simulink model "consigna_5_1"  (R2024b)
settings: Solver=VariableStepAuto  StartTime=0.0  StopTime=1  MaxStep=1e-4  RelTol=1e-3
InitFcn:
  | parametros
undefined symbols (not defined in the file or in its folder): alpha_cu, b_eq, b_l, b_m, C_ts, J_eq, J_l, J_m, k_l, L_d, L_ls, L_q, lambda_m, P_p, r, R_s_40, R_ts_amb, Temp_s_ref
(part 2 of 3)

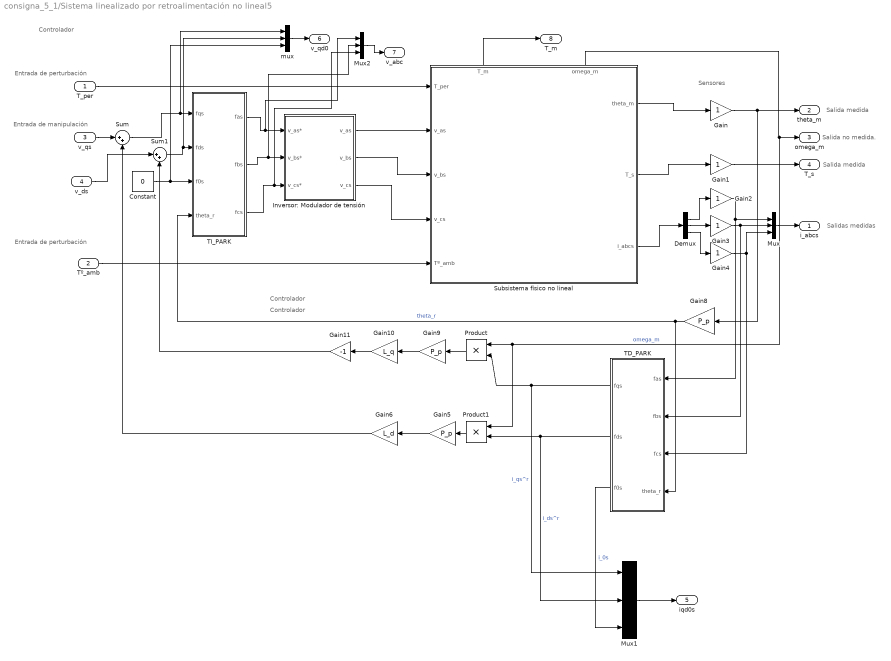
== system consigna_5_1/Sistema linealizado por retroalimentación no lineal5 ==
  note: Entrada de perturbación
  note: Entrada de manipulación
  note: Entrada de perturbación
  note: Controlador
  note: Salida medida
  note: Controlador
  note: Sensores
  note: Salida medida
  note: Salidas medidas
  note: Salida no medida.
  note: Controlador
  T_per : Inport
  Tº_amb : Inport  Port=2
  v_qs : Inport  Port=3
  v_ds : Inport  Port=4
  Constant : Constant  Value=0
  Demux : Demux  Outputs=3
  Gain{,1..4} (5 alike) : Gain
  Gain10 : Gain  Gain=L_q
  Gain11 : Gain  Gain=-1
  Gain5 : Gain  Gain=P_p
  Gain6 : Gain  Gain=L_d
  Gain8 : Gain  Gain=P_p
  Gain9 : Gain  Gain=P_p
  Inversor: Modulador de tensión : Subsystem
  Mux : Mux  Inputs=3
  Mux1 : Mux  Inputs=3
  Mux2 : Mux  Inputs=3
  Product : Product
  Product1 : Product
  Subsistema físico no lineal : Subsystem
      settings: PortSchema="{\"entries\":[{\"content\":{\"sides\":[{\"content\":{\"connectorIds\":[\"In1\",\"In2\",\"In3\",\"In4\",\"In5\"]},\"type\":\"ConnectorPlacement.EquallySpacedRectSide\",\"uuid\":\"67117692-d9ee-40bf-88b2-d8f6a60dc3b5\"},{\"content\":{\"connectorIds\":[\"Out1\",\"Out2\",\"Out3\"],\"side\":\"RIGHT\"},\"type\":\"ConnectorPlacement.EquallySpacedRectSide\",\"uuid\":\"ca2dbe86-e86f-47c7-8eac-1e82e6a5dbc0\"},{\"content\":{\"connectorIds\":[\"Out4\",\"Out5\"],\"side\":\"TOP\"},\"type\":\"ConnectorPlacement.EquallySpacedRectSide\",\"uuid\":\"fbd4a5c3-5162-48dd-8002-932f8e6631f6\"}]},\"type\":\"ConnectorPlacement.EquallySpacedConnector\",\"uuid\":\"e55c07f0-88b9-4508-920f-2bf50421126b\"}],\"packageUris\":[\"http://schema.mathworks.com/mf0/Connector/R2020b\"],\"version\":\"1.0\"}"
  Sum : Sum  Inputs=|++
  Sum1 : Sum  Inputs=|++
  TD_PARK : MATLAB Function  TreatAsAtomicUnit=on
  TI_PARK : MATLAB Function  TreatAsAtomicUnit=on
  mux : Mux  Inputs=3
  i_abcs : Outport
  theta_m : Outport  Port=2
  omega_m : Outport  Port=3
  T_s : Outport  Port=4
  iqd0s : Outport  Port=5
  v_qd0 : Outport  Port=6
  v_abc : Outport  Port=7
  T_m : Outport  Port=8
  wires:
  T_per/1 -> Subsistema físico no lineal/1(T_per)
  Subsistema físico no lineal/2(T_s) -> Gain1/1
  Subsistema físico no lineal/1(theta_m) -> Gain/1
  Tº_amb/1 -> Subsistema físico no lineal/5(Tº_amb)
  Demux/3 -> Gain4/1
  Demux/1 -> Gain2/1
  Gain2/1 -> Mux/1, TD_PARK/1(fas)
  Gain3/1 -> Mux/2, TD_PARK/2(fbs)
  Gain4/1 -> Mux/3, TD_PARK/3(fcs)
  Mux/1 -> i_abcs/1
  Gain/1 -> Gain8/1, theta_m/1
  Subsistema físico no lineal/5(omega_m) -> omega_m/1, Product1/1, Product/1  "omega_m"
  Gain1/1 -> T_s/1
  Gain8/1 -> TI_PARK/4(theta_r), TD_PARK/4(theta_r)  "theta_r"
  TD_PARK/1(fqs) -> Mux1/1, Product/2  "i_qs^r"
  Product/1 -> Gain9/1
  Gain9/1 -> Gain10/1
  Gain10/1 -> Gain11/1
  Constant/1 -> TI_PARK/3(f0s), mux/3
  Inversor: Modulador de tensión/1(v_as) -> Subsistema físico no lineal/2(v_as)
  Inversor: Modulador de tensión/2(v_bs) -> Subsistema físico no lineal/3(v_bs)
  Inversor: Modulador de tensión/3(v_cs) -> Subsistema físico no lineal/4(v_cs)
  TI_PARK/1(fas) -> Mux2/1, Inversor: Modulador de tensión/1(v_as*)
  TI_PARK/2(fbs) -> Mux2/2, Inversor: Modulador de tensión/2(v_bs*)
  TI_PARK/3(fcs) -> Mux2/3, Inversor: Modulador de tensión/3(v_cs*)
  TD_PARK/2(fds) -> Mux1/2, Product1/2  "i_ds^r"
  TD_PARK/3(f0s) -> Mux1/3  "i_0s"
  v_qs/1 -> Sum/1
  Sum/1 -> mux/1, TI_PARK/1(fqs)
  Product1/1 -> Gain5/1
  Gain5/1 -> Gain6/1
  Gain6/1 -> Sum/2
  Mux1/1 -> iqd0s/1
  mux/1 -> v_qd0/1
  Mux2/1 -> v_abc/1
  Subsistema físico no lineal/4(T_m) -> T_m/1
  Subsistema físico no lineal/3(i_abcs) -> Demux/1
  Demux/2 -> Gain3/1
  Gain11/1 -> Sum1/2
  v_ds/1 -> Sum1/1
  Sum1/1 -> mux/2, TI_PARK/2(fds)

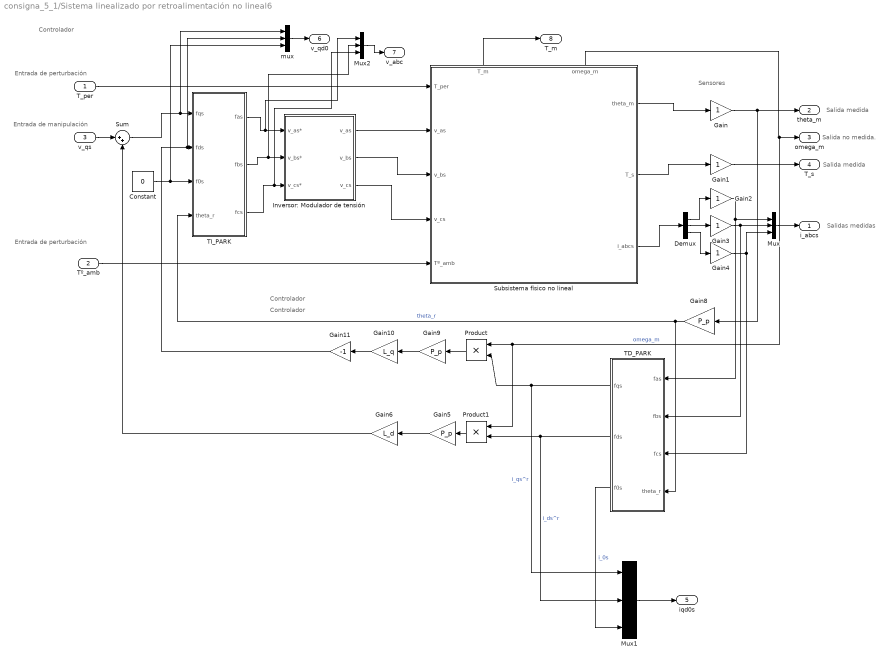
== system consigna_5_1/Sistema linealizado por retroalimentación no lineal6 ==
  note: Entrada de perturbación
  note: Entrada de manipulación
  note: Entrada de perturbación
  note: Controlador
  note: Salida medida
  note: Controlador
  note: Sensores
  note: Salida medida
  note: Salidas medidas
  note: Salida no medida.
  note: Controlador
  T_per : Inport
  Tº_amb : Inport  Port=2
  v_qs : Inport  Port=3
  Constant : Constant  Value=0
  Demux : Demux  Outputs=3
  Gain{,1..4} (5 alike) : Gain
  Gain10 : Gain  Gain=L_q
  Gain11 : Gain  Gain=-1
  Gain5 : Gain  Gain=P_p
  Gain6 : Gain  Gain=L_d
  Gain8 : Gain  Gain=P_p
  Gain9 : Gain  Gain=P_p
  Inversor: Modulador de tensión : Subsystem
  Mux : Mux  Inputs=3
  Mux1 : Mux  Inputs=3
  Mux2 : Mux  Inputs=3
  Product : Product
  Product1 : Product
  Subsistema físico no lineal : Subsystem
      settings: PortSchema="{\"entries\":[{\"content\":{\"sides\":[{\"content\":{\"connectorIds\":[\"In1\",\"In2\",\"In3\",\"In4\",\"In5\"]},\"type\":\"ConnectorPlacement.EquallySpacedRectSide\",\"uuid\":\"67117692-d9ee-40bf-88b2-d8f6a60dc3b5\"},{\"content\":{\"connectorIds\":[\"Out1\",\"Out2\",\"Out3\"],\"side\":\"RIGHT\"},\"type\":\"ConnectorPlacement.EquallySpacedRectSide\",\"uuid\":\"ca2dbe86-e86f-47c7-8eac-1e82e6a5dbc0\"},{\"content\":{\"connectorIds\":[\"Out4\",\"Out5\"],\"side\":\"TOP\"},\"type\":\"ConnectorPlacement.EquallySpacedRectSide\",\"uuid\":\"fbd4a5c3-5162-48dd-8002-932f8e6631f6\"}]},\"type\":\"ConnectorPlacement.EquallySpacedConnector\",\"uuid\":\"e55c07f0-88b9-4508-920f-2bf50421126b\"}],\"packageUris\":[\"http://schema.mathworks.com/mf0/Connector/R2020b\"],\"version\":\"1.0\"}"
  Sum : Sum  Inputs=|++
  TD_PARK : MATLAB Function  TreatAsAtomicUnit=on
  TI_PARK : MATLAB Function  TreatAsAtomicUnit=on
  mux : Mux  Inputs=3
  i_abcs : Outport
  theta_m : Outport  Port=2
  omega_m : Outport  Port=3
  T_s : Outport  Port=4
  iqd0s : Outport  Port=5
  v_qd0 : Outport  Port=6
  v_abc : Outport  Port=7
  T_m : Outport  Port=8
  wires:
  T_per/1 -> Subsistema físico no lineal/1(T_per)
  Subsistema físico no lineal/2(T_s) -> Gain1/1
  Subsistema físico no lineal/1(theta_m) -> Gain/1
  Tº_amb/1 -> Subsistema físico no lineal/5(Tº_amb)
  Demux/3 -> Gain4/1
  Demux/1 -> Gain2/1
  Gain2/1 -> Mux/1, TD_PARK/1(fas)
  Gain3/1 -> Mux/2, TD_PARK/2(fbs)
  Gain4/1 -> Mux/3, TD_PARK/3(fcs)
  Mux/1 -> i_abcs/1
  Gain/1 -> Gain8/1, theta_m/1
  Subsistema físico no lineal/5(omega_m) -> omega_m/1, Product1/1, Product/1  "omega_m"
  Gain1/1 -> T_s/1
  Gain8/1 -> TI_PARK/4(theta_r), TD_PARK/4(theta_r)  "theta_r"
  TD_PARK/1(fqs) -> Mux1/1, Product/2  "i_qs^r"
  Product/1 -> Gain9/1
  Gain9/1 -> Gain10/1
  Gain11/1 -> mux/2, TI_PARK/2(fds)
  Gain10/1 -> Gain11/1
  Constant/1 -> TI_PARK/3(f0s), mux/3
  Inversor: Modulador de tensión/1(v_as) -> Subsistema físico no lineal/2(v_as)
  Inversor: Modulador de tensión/2(v_bs) -> Subsistema físico no lineal/3(v_bs)
  Inversor: Modulador de tensión/3(v_cs) -> Subsistema físico no lineal/4(v_cs)
  TI_PARK/1(fas) -> Mux2/1, Inversor: Modulador de tensión/1(v_as*)
  TI_PARK/2(fbs) -> Mux2/2, Inversor: Modulador de tensión/2(v_bs*)
  TI_PARK/3(fcs) -> Mux2/3, Inversor: Modulador de tensión/3(v_cs*)
  TD_PARK/2(fds) -> Mux1/2, Product1/2  "i_ds^r"
  TD_PARK/3(f0s) -> Mux1/3  "i_0s"
  v_qs/1 -> Sum/1
  Sum/1 -> mux/1, TI_PARK/1(fqs)
  Product1/1 -> Gain5/1
  Gain5/1 -> Gain6/1
  Gain6/1 -> Sum/2
  Mux1/1 -> iqd0s/1
  mux/1 -> v_qd0/1
  Mux2/1 -> v_abc/1
  Subsistema físico no lineal/4(T_m) -> T_m/1
  Subsistema físico no lineal/3(i_abcs) -> Demux/1
  Demux/2 -> Gain3/1

== system consigna_5_1/Sistema completo/Subsistema físico no lineal ==
  note: Retroalimentación natural del torque gravitacional
  Tº_amb : Inport
  v_as : Inport  Port=2
  v_bs : Inport  Port=3
  v_cs : Inport  Port=4
  T_per : Inport  Port=5
  Gain : Gain  Gain=P_p
  Gain1 : Gain  Gain=1/r
  Gain2 : Gain  Gain=k_l
  Mux : Mux  Inputs=3
  Sin : Trigonometry
  Subsistema electromagnético : Subsystem
      settings: PortSchema="{\"entries\":[{\"content\":{\"sides\":[{\"content\":{\"connectorIds\":[\"In1\",\"In2\",\"In3\",\"In4\"]},\"type\":\"ConnectorPlacement.EquallySpacedRectSide\",\"uuid\":\"c9fae60f-a644-4c7d-9a50-e330e891aba8\"},{\"content\":{\"connectorIds\":[\"Out1\",\"Out2\",\"Out3\",\"Out4\"],\"side\":\"RIGHT\"},\"type\":\"ConnectorPlacement.EquallySpacedRectSide\",\"uuid\":\"1bd25713-f5e9-4106-83eb-fb9f8a30d88e\"},{\"content\":{\"connectorIds\":[\"In5\"],\"side\":\"TOP\"},\"type\":\"ConnectorPlacement.EquallySpacedRectSide\",\"uuid\":\"c2f005dd-e04f-426d-b804-ce475aa5422d\"}]},\"type\":\"ConnectorPlacement.EquallySpacedConnector\",\"uuid\":\"9bdc4406-fcef-47cb-a5c0-d4f33f547a91\"}],\"packageUris\":[\"http://schema.mathworks.com/mf0/Connector/R2020b\"],\"version\":\"1.0\"}"
  Subsistema mecánico completo : Subsystem
  Subsistema térmico : Subsystem
  Sum : Sum  Inputs=++|
  TD_PARK : MATLAB Function  TreatAsAtomicUnit=on
  TI_PARK : MATLAB Function  TreatAsAtomicUnit=on
  theta_m : Outport
  omega_m : Outport  Port=2
  T_s : Outport  Port=3
  i_abcs : Outport  Port=4
  wires:
  Subsistema electromagnético/4(T_m) -> Subsistema mecánico completo/1(T_m)
  Subsistema electromagnético/3(i_0s) -> Subsistema térmico/3(i_0s^r), TI_PARK/3(f0s)
  Subsistema mecánico completo/2(omega_m(t)) -> Subsistema electromagnético/5(omega_m), omega_m/1
  Subsistema electromagnético/1(i_qs^r) -> Subsistema térmico/1(i_qs^r), TI_PARK/1(fqs)
  Subsistema electromagnético/2(i_ds^r) -> Subsistema térmico/2(i_ds^r), TI_PARK/2(fds)
  Sum/1 -> Subsistema mecánico completo/2(T_l)  "T_l"
  TD_PARK/1(fqs) -> Subsistema electromagnético/1(v_qs^r)
  Subsistema mecánico completo/1(theta_m(t)) -> theta_m/1, Gain1/1, Gain/1
  Tº_amb/1 -> Subsistema térmico/4(Tº_amb)
  Mux/1 -> i_abcs/1
  TI_PARK/1(fas) -> Mux/1
  TI_PARK/2(fbs) -> Mux/2
  TI_PARK/3(fcs) -> Mux/3
  v_as/1 -> TD_PARK/1(fas)
  v_cs/1 -> TD_PARK/3(fcs)
  Gain/1 -> TI_PARK/4(theta_r), TD_PARK/4(theta_r)
  v_bs/1 -> TD_PARK/2(fbs)
  Gain1/1 -> Sin/1
  Sin/1 -> Gain2/1
  Gain2/1 -> Sum/1
  T_per/1 -> Sum/2
  TD_PARK/2(fds) -> Subsistema electromagnético/2(v_ds^r)
  TD_PARK/3(f0s) -> Subsistema electromagnético/3(v_0s)
  Subsistema térmico/1(r_s) -> Subsistema electromagnético/4(r_s)
  Subsistema térmico/2(T_s) -> T_s/1

== system consigna_5_1/Sistema linealizado por retroalimentación no lineal1/Inversor: Modulador de tensión ==
  v_as* : Inport
  v_bs* : Inport  Port=2
  v_cs* : Inport  Port=3
  Gain5 : Gain
  Gain6 : Gain
  Gain7 : Gain
  v_as : Outport
  v_bs : Outport  Port=2
  v_cs : Outport  Port=3
  wires:
  v_as*/1 -> Gain5/1
  Gain5/1 -> v_as/1
  v_cs*/1 -> Gain7/1
  v_bs*/1 -> Gain6/1
  Gain7/1 -> v_cs/1
  Gain6/1 -> v_bs/1

== system consigna_5_1/Sistema linealizado por retroalimentación no lineal1/Subsistema físico no lineal ==
  note: Retroalimentación natural del torque gravitacional
  T_per : Inport
  v_as : Inport  Port=2
  v_bs : Inport  Port=3
  v_cs : Inport  Port=4
  Tº_amb : Inport  Port=5
  Gain : Gain  Gain=P_p
  Gain1 : Gain  Gain=1/r
  Gain2 : Gain  Gain=k_l
  Mux : Mux  Inputs=3
  Scope : Scope
  Sin : Trigonometry
  Subsistema electromagnético : Subsystem
      settings: PortSchema="{\"entries\":[{\"content\":{\"sides\":[{\"content\":{\"connectorIds\":[\"In1\",\"In2\",\"In3\",\"In4\"]},\"type\":\"ConnectorPlacement.EquallySpacedRectSide\",\"uuid\":\"c9fae60f-a644-4c7d-9a50-e330e891aba8\"},{\"content\":{\"connectorIds\":[\"Out1\",\"Out2\",\"Out3\",\"Out4\"],\"side\":\"RIGHT\"},\"type\":\"ConnectorPlacement.EquallySpacedRectSide\",\"uuid\":\"1bd25713-f5e9-4106-83eb-fb9f8a30d88e\"},{\"content\":{\"connectorIds\":[\"In5\"],\"side\":\"TOP\"},\"type\":\"ConnectorPlacement.EquallySpacedRectSide\",\"uuid\":\"c2f005dd-e04f-426d-b804-ce475aa5422d\"}]},\"type\":\"ConnectorPlacement.EquallySpacedConnector\",\"uuid\":\"9bdc4406-fcef-47cb-a5c0-d4f33f547a91\"}],\"packageUris\":[\"http://schema.mathworks.com/mf0/Connector/R2020b\"],\"version\":\"1.0\"}"
  Subsistema mecánico completo : Subsystem
  Subsistema térmico : Subsystem
  Sum : Sum  Inputs=++|
  TD_PARK : MATLAB Function  TreatAsAtomicUnit=on
  TI_PARK : MATLAB Function  TreatAsAtomicUnit=on
  theta_m : Outport
  T_s : Outport  Port=2
  i_abcs : Outport  Port=3
  T_m : Outport  Port=4
  omega_m : Outport  Port=5
  wires:
  Subsistema electromagnético/4(T_m) -> T_m/1, Subsistema mecánico completo/1(T_m)
  Subsistema electromagnético/3(i_0s) -> Subsistema térmico/3(i_0s^r), TI_PARK/3(f0s)
  Subsistema mecánico completo/2(omega_m(t)) -> Subsistema electromagnético/5(omega_m), Scope/1, omega_m/1
  Subsistema electromagnético/1(i_qs^r) -> Subsistema térmico/1(i_qs^r), TI_PARK/1(fqs)
  Subsistema electromagnético/2(i_ds^r) -> Subsistema térmico/2(i_ds^r), TI_PARK/2(fds)
  Sum/1 -> Subsistema mecánico completo/2(T_l)  "T_l"
  TD_PARK/1(fqs) -> Subsistema electromagnético/1(v_qs^r)
  Tº_amb/1 -> Subsistema térmico/4(Tº_amb)
  Mux/1 -> i_abcs/1
  TI_PARK/1(fas) -> Mux/1
  TI_PARK/2(fbs) -> Mux/2
  TI_PARK/3(fcs) -> Mux/3
  v_as/1 -> TD_PARK/1(fas)
  v_cs/1 -> TD_PARK/3(fcs)
  Gain/1 -> TI_PARK/4(theta_r), TD_PARK/4(theta_r)
  v_bs/1 -> TD_PARK/2(fbs)
  Gain1/1 -> Sin/1
  Sin/1 -> Gain2/1
  Gain2/1 -> Sum/1
  T_per/1 -> Sum/2
  TD_PARK/2(fds) -> Subsistema electromagnético/2(v_ds^r)
  TD_PARK/3(f0s) -> Subsistema electromagnético/3(v_0s)
  Subsistema térmico/1(r_s) -> Subsistema electromagnético/4(r_s)
  Subsistema térmico/2(T_s) -> T_s/1
  Subsistema mecánico completo/1(theta_m(t)) -> theta_m/1, Gain1/1, Gain/1

== system consigna_5_1/Sistema linealizado por retroalimentación no lineal2/Inversor: Modulador de tensión ==
  v_as* : Inport
  v_bs* : Inport  Port=2
  v_cs* : Inport  Port=3
  Gain5 : Gain
  Gain6 : Gain
  Gain7 : Gain
  v_as : Outport
  v_bs : Outport  Port=2
  v_cs : Outport  Port=3
  wires:
  v_as*/1 -> Gain5/1
  Gain5/1 -> v_as/1
  v_cs*/1 -> Gain7/1
  v_bs*/1 -> Gain6/1
  Gain7/1 -> v_cs/1
  Gain6/1 -> v_bs/1

== system consigna_5_1/Sistema linealizado por retroalimentación no lineal2/Subsistema físico no lineal ==
  note: Retroalimentación natural del torque gravitacional
  T_per : Inport
  v_as : Inport  Port=2
  v_bs : Inport  Port=3
  v_cs : Inport  Port=4
  Tº_amb : Inport  Port=5
  Gain : Gain  Gain=P_p
  Gain1 : Gain  Gain=1/r
  Gain2 : Gain  Gain=k_l
  Mux : Mux  Inputs=3
  Scope : Scope
  Sin : Trigonometry
  Subsistema electromagnético : Subsystem
      settings: PortSchema="{\"entries\":[{\"content\":{\"sides\":[{\"content\":{\"connectorIds\":[\"In1\",\"In2\",\"In3\",\"In4\"]},\"type\":\"ConnectorPlacement.EquallySpacedRectSide\",\"uuid\":\"c9fae60f-a644-4c7d-9a50-e330e891aba8\"},{\"content\":{\"connectorIds\":[\"Out1\",\"Out2\",\"Out3\",\"Out4\"],\"side\":\"RIGHT\"},\"type\":\"ConnectorPlacement.EquallySpacedRectSide\",\"uuid\":\"1bd25713-f5e9-4106-83eb-fb9f8a30d88e\"},{\"content\":{\"connectorIds\":[\"In5\"],\"side\":\"TOP\"},\"type\":\"ConnectorPlacement.EquallySpacedRectSide\",\"uuid\":\"c2f005dd-e04f-426d-b804-ce475aa5422d\"}]},\"type\":\"ConnectorPlacement.EquallySpacedConnector\",\"uuid\":\"9bdc4406-fcef-47cb-a5c0-d4f33f547a91\"}],\"packageUris\":[\"http://schema.mathworks.com/mf0/Connector/R2020b\"],\"version\":\"1.0\"}"
  Subsistema mecánico completo : Subsystem
  Subsistema térmico : Subsystem
  Sum : Sum  Inputs=++|
  TD_PARK : MATLAB Function  TreatAsAtomicUnit=on
  TI_PARK : MATLAB Function  TreatAsAtomicUnit=on
  theta_m : Outport
  T_s : Outport  Port=2
  i_abcs : Outport  Port=3
  T_m : Outport  Port=4
  omega_m : Outport  Port=5
  wires:
  Subsistema electromagnético/4(T_m) -> T_m/1, Subsistema mecánico completo/1(T_m)
  Subsistema electromagnético/3(i_0s) -> Subsistema térmico/3(i_0s^r), TI_PARK/3(f0s)
  Subsistema mecánico completo/2(omega_m(t)) -> Subsistema electromagnético/5(omega_m), Scope/1, omega_m/1
  Subsistema electromagnético/1(i_qs^r) -> Subsistema térmico/1(i_qs^r), TI_PARK/1(fqs)
  Subsistema electromagnético/2(i_ds^r) -> Subsistema térmico/2(i_ds^r), TI_PARK/2(fds)
  Sum/1 -> Subsistema mecánico completo/2(T_l)  "T_l"
  TD_PARK/1(fqs) -> Subsistema electromagnético/1(v_qs^r)
  Tº_amb/1 -> Subsistema térmico/4(Tº_amb)
  Mux/1 -> i_abcs/1
  TI_PARK/1(fas) -> Mux/1
  TI_PARK/2(fbs) -> Mux/2
  TI_PARK/3(fcs) -> Mux/3
  v_as/1 -> TD_PARK/1(fas)
  v_cs/1 -> TD_PARK/3(fcs)
  Gain/1 -> TI_PARK/4(theta_r), TD_PARK/4(theta_r)
  v_bs/1 -> TD_PARK/2(fbs)
  Gain1/1 -> Sin/1
  Sin/1 -> Gain2/1
  Gain2/1 -> Sum/1
  T_per/1 -> Sum/2
  TD_PARK/2(fds) -> Subsistema electromagnético/2(v_ds^r)
  TD_PARK/3(f0s) -> Subsistema electromagnético/3(v_0s)
  Subsistema térmico/1(r_s) -> Subsistema electromagnético/4(r_s)
  Subsistema térmico/2(T_s) -> T_s/1
  Subsistema mecánico completo/1(theta_m(t)) -> theta_m/1, Gain1/1, Gain/1

== system consigna_5_1/Sistema linealizado por retroalimentación no lineal3/Inversor: Modulador de tensión ==
  v_as* : Inport
  v_bs* : Inport  Port=2
  v_cs* : Inport  Port=3
  Gain5 : Gain
  Gain6 : Gain
  Gain7 : Gain
  v_as : Outport
  v_bs : Outport  Port=2
  v_cs : Outport  Port=3
  wires:
  v_as*/1 -> Gain5/1
  Gain5/1 -> v_as/1
  v_cs*/1 -> Gain7/1
  v_bs*/1 -> Gain6/1
  Gain7/1 -> v_cs/1
  Gain6/1 -> v_bs/1

== system consigna_5_1/Sistema linealizado por retroalimentación no lineal3/Subsistema físico no lineal ==
  note: Retroalimentación natural del torque gravitacional
  T_per : Inport
  v_as : Inport  Port=2
  v_bs : Inport  Port=3
  v_cs : Inport  Port=4
  Tº_amb : Inport  Port=5
  Gain : Gain  Gain=P_p
  Gain1 : Gain  Gain=1/r
  Gain2 : Gain  Gain=k_l
  Mux : Mux  Inputs=3
  Scope : Scope
  Sin : Trigonometry
  Subsistema electromagnético : Subsystem
      settings: PortSchema="{\"entries\":[{\"content\":{\"sides\":[{\"content\":{\"connectorIds\":[\"In1\",\"In2\",\"In3\",\"In4\"]},\"type\":\"ConnectorPlacement.EquallySpacedRectSide\",\"uuid\":\"c9fae60f-a644-4c7d-9a50-e330e891aba8\"},{\"content\":{\"connectorIds\":[\"Out1\",\"Out2\",\"Out3\",\"Out4\"],\"side\":\"RIGHT\"},\"type\":\"ConnectorPlacement.EquallySpacedRectSide\",\"uuid\":\"1bd25713-f5e9-4106-83eb-fb9f8a30d88e\"},{\"content\":{\"connectorIds\":[\"In5\"],\"side\":\"TOP\"},\"type\":\"ConnectorPlacement.EquallySpacedRectSide\",\"uuid\":\"c2f005dd-e04f-426d-b804-ce475aa5422d\"}]},\"type\":\"ConnectorPlacement.EquallySpacedConnector\",\"uuid\":\"9bdc4406-fcef-47cb-a5c0-d4f33f547a91\"}],\"packageUris\":[\"http://schema.mathworks.com/mf0/Connector/R2020b\"],\"version\":\"1.0\"}"
  Subsistema mecánico completo : Subsystem
  Subsistema térmico : Subsystem
  Sum : Sum  Inputs=++|
  TD_PARK : MATLAB Function  TreatAsAtomicUnit=on
  TI_PARK : MATLAB Function  TreatAsAtomicUnit=on
  theta_m : Outport
  T_s : Outport  Port=2
  i_abcs : Outport  Port=3
  T_m : Outport  Port=4
  omega_m : Outport  Port=5
  wires:
  Subsistema electromagnético/4(T_m) -> T_m/1, Subsistema mecánico completo/1(T_m)
  Subsistema electromagnético/3(i_0s) -> Subsistema térmico/3(i_0s^r), TI_PARK/3(f0s)
  Subsistema mecánico completo/2(omega_m(t)) -> Subsistema electromagnético/5(omega_m), Scope/1, omega_m/1
  Subsistema electromagnético/1(i_qs^r) -> Subsistema térmico/1(i_qs^r), TI_PARK/1(fqs)
  Subsistema electromagnético/2(i_ds^r) -> Subsistema térmico/2(i_ds^r), TI_PARK/2(fds)
  Sum/1 -> Subsistema mecánico completo/2(T_l)  "T_l"
  TD_PARK/1(fqs) -> Subsistema electromagnético/1(v_qs^r)
  Tº_amb/1 -> Subsistema térmico/4(Tº_amb)
  Mux/1 -> i_abcs/1
  TI_PARK/1(fas) -> Mux/1
  TI_PARK/2(fbs) -> Mux/2
  TI_PARK/3(fcs) -> Mux/3
  v_as/1 -> TD_PARK/1(fas)
  v_cs/1 -> TD_PARK/3(fcs)
  Gain/1 -> TI_PARK/4(theta_r), TD_PARK/4(theta_r)
  v_bs/1 -> TD_PARK/2(fbs)
  Gain1/1 -> Sin/1
  Sin/1 -> Gain2/1
  Gain2/1 -> Sum/1
  T_per/1 -> Sum/2
  TD_PARK/2(fds) -> Subsistema electromagnético/2(v_ds^r)
  TD_PARK/3(f0s) -> Subsistema electromagnético/3(v_0s)
  Subsistema térmico/1(r_s) -> Subsistema electromagnético/4(r_s)
  Subsistema térmico/2(T_s) -> T_s/1
  Subsistema mecánico completo/1(theta_m(t)) -> theta_m/1, Gain1/1, Gain/1

== system consigna_5_1/Sistema linealizado por retroalimentación no lineal4/Inversor: Modulador de tensión ==
  v_as* : Inport
  v_bs* : Inport  Port=2
  v_cs* : Inport  Port=3
  Gain5 : Gain
  Gain6 : Gain
  Gain7 : Gain
  v_as : Outport
  v_bs : Outport  Port=2
  v_cs : Outport  Port=3
  wires:
  v_as*/1 -> Gain5/1
  Gain5/1 -> v_as/1
  v_cs*/1 -> Gain7/1
  v_bs*/1 -> Gain6/1
  Gain7/1 -> v_cs/1
  Gain6/1 -> v_bs/1

== system consigna_5_1/Sistema linealizado por retroalimentación no lineal4/Subsistema físico no lineal ==
  note: Retroalimentación natural del torque gravitacional
  T_per : Inport
  v_as : Inport  Port=2
  v_bs : Inport  Port=3
  v_cs : Inport  Port=4
  Tº_amb : Inport  Port=5
  Gain : Gain  Gain=P_p
  Gain1 : Gain  Gain=1/r
  Gain2 : Gain  Gain=k_l
  Mux : Mux  Inputs=3
  Scope : Scope
  Sin : Trigonometry
  Subsistema electromagnético : Subsystem
      settings: PortSchema="{\"entries\":[{\"content\":{\"sides\":[{\"content\":{\"connectorIds\":[\"In1\",\"In2\",\"In3\",\"In4\"]},\"type\":\"ConnectorPlacement.EquallySpacedRectSide\",\"uuid\":\"c9fae60f-a644-4c7d-9a50-e330e891aba8\"},{\"content\":{\"connectorIds\":[\"Out1\",\"Out2\",\"Out3\",\"Out4\"],\"side\":\"RIGHT\"},\"type\":\"ConnectorPlacement.EquallySpacedRectSide\",\"uuid\":\"1bd25713-f5e9-4106-83eb-fb9f8a30d88e\"},{\"content\":{\"connectorIds\":[\"In5\"],\"side\":\"TOP\"},\"type\":\"ConnectorPlacement.EquallySpacedRectSide\",\"uuid\":\"c2f005dd-e04f-426d-b804-ce475aa5422d\"}]},\"type\":\"ConnectorPlacement.EquallySpacedConnector\",\"uuid\":\"9bdc4406-fcef-47cb-a5c0-d4f33f547a91\"}],\"packageUris\":[\"http://schema.mathworks.com/mf0/Connector/R2020b\"],\"version\":\"1.0\"}"
  Subsistema mecánico completo : Subsystem
  Subsistema térmico : Subsystem
  Sum : Sum  Inputs=++|
  TD_PARK : MATLAB Function  TreatAsAtomicUnit=on
  TI_PARK : MATLAB Function  TreatAsAtomicUnit=on
  theta_m : Outport
  T_s : Outport  Port=2
  i_abcs : Outport  Port=3
  T_m : Outport  Port=4
  omega_m : Outport  Port=5
  wires:
  Subsistema electromagnético/4(T_m) -> T_m/1, Subsistema mecánico completo/1(T_m)
  Subsistema electromagnético/3(i_0s) -> Subsistema térmico/3(i_0s^r), TI_PARK/3(f0s)
  Subsistema mecánico completo/2(omega_m(t)) -> Subsistema electromagnético/5(omega_m), Scope/1, omega_m/1
  Subsistema electromagnético/1(i_qs^r) -> Subsistema térmico/1(i_qs^r), TI_PARK/1(fqs)
  Subsistema electromagnético/2(i_ds^r) -> Subsistema térmico/2(i_ds^r), TI_PARK/2(fds)
  Sum/1 -> Subsistema mecánico completo/2(T_l)  "T_l"
  TD_PARK/1(fqs) -> Subsistema electromagnético/1(v_qs^r)
  Tº_amb/1 -> Subsistema térmico/4(Tº_amb)
  Mux/1 -> i_abcs/1
  TI_PARK/1(fas) -> Mux/1
  TI_PARK/2(fbs) -> Mux/2
  TI_PARK/3(fcs) -> Mux/3
  v_as/1 -> TD_PARK/1(fas)
  v_cs/1 -> TD_PARK/3(fcs)
  Gain/1 -> TI_PARK/4(theta_r), TD_PARK/4(theta_r)
  v_bs/1 -> TD_PARK/2(fbs)
  Gain1/1 -> Sin/1
  Sin/1 -> Gain2/1
  Gain2/1 -> Sum/1
  T_per/1 -> Sum/2
  TD_PARK/2(fds) -> Subsistema electromagnético/2(v_ds^r)
  TD_PARK/3(f0s) -> Subsistema electromagnético/3(v_0s)
  Subsistema térmico/1(r_s) -> Subsistema electromagnético/4(r_s)
  Subsistema térmico/2(T_s) -> T_s/1
  Subsistema mecánico completo/1(theta_m(t)) -> theta_m/1, Gain1/1, Gain/1

== system consigna_5_1/Sistema linealizado por retroalimentación no lineal5/Inversor: Modulador de tensión ==
  v_as* : Inport
  v_bs* : Inport  Port=2
  v_cs* : Inport  Port=3
  Gain5 : Gain
  Gain6 : Gain
  Gain7 : Gain
  v_as : Outport
  v_bs : Outport  Port=2
  v_cs : Outport  Port=3
  wires:
  v_as*/1 -> Gain5/1
  Gain5/1 -> v_as/1
  v_cs*/1 -> Gain7/1
  v_bs*/1 -> Gain6/1
  Gain7/1 -> v_cs/1
  Gain6/1 -> v_bs/1

== system consigna_5_1/Sistema linealizado por retroalimentación no lineal5/Subsistema físico no lineal ==
  note: Retroalimentación natural del torque gravitacional
  T_per : Inport
  v_as : Inport  Port=2
  v_bs : Inport  Port=3
  v_cs : Inport  Port=4
  Tº_amb : Inport  Port=5
  Gain : Gain  Gain=P_p
  Gain1 : Gain  Gain=1/r
  Gain2 : Gain  Gain=k_l
  Mux : Mux  Inputs=3
  Scope : Scope
  Sin : Trigonometry
  Subsistema electromagnético : Subsystem
      settings: PortSchema="{\"entries\":[{\"content\":{\"sides\":[{\"content\":{\"connectorIds\":[\"In1\",\"In2\",\"In3\",\"In4\"]},\"type\":\"ConnectorPlacement.EquallySpacedRectSide\",\"uuid\":\"c9fae60f-a644-4c7d-9a50-e330e891aba8\"},{\"content\":{\"connectorIds\":[\"Out1\",\"Out2\",\"Out3\",\"Out4\"],\"side\":\"RIGHT\"},\"type\":\"ConnectorPlacement.EquallySpacedRectSide\",\"uuid\":\"1bd25713-f5e9-4106-83eb-fb9f8a30d88e\"},{\"content\":{\"connectorIds\":[\"In5\"],\"side\":\"TOP\"},\"type\":\"ConnectorPlacement.EquallySpacedRectSide\",\"uuid\":\"c2f005dd-e04f-426d-b804-ce475aa5422d\"}]},\"type\":\"ConnectorPlacement.EquallySpacedConnector\",\"uuid\":\"9bdc4406-fcef-47cb-a5c0-d4f33f547a91\"}],\"packageUris\":[\"http://schema.mathworks.com/mf0/Connector/R2020b\"],\"version\":\"1.0\"}"
  Subsistema mecánico completo : Subsystem
  Subsistema térmico : Subsystem
  Sum : Sum  Inputs=++|
  TD_PARK : MATLAB Function  TreatAsAtomicUnit=on
  TI_PARK : MATLAB Function  TreatAsAtomicUnit=on
  theta_m : Outport
  T_s : Outport  Port=2
  i_abcs : Outport  Port=3
  T_m : Outport  Port=4
  omega_m : Outport  Port=5
  wires:
  Subsistema electromagnético/4(T_m) -> T_m/1, Subsistema mecánico completo/1(T_m)
  Subsistema electromagnético/3(i_0s) -> Subsistema térmico/3(i_0s^r), TI_PARK/3(f0s)
  Subsistema mecánico completo/2(omega_m(t)) -> Subsistema electromagnético/5(omega_m), Scope/1, omega_m/1
  Subsistema electromagnético/1(i_qs^r) -> Subsistema térmico/1(i_qs^r), TI_PARK/1(fqs)
  Subsistema electromagnético/2(i_ds^r) -> Subsistema térmico/2(i_ds^r), TI_PARK/2(fds)
  Sum/1 -> Subsistema mecánico completo/2(T_l)  "T_l"
  TD_PARK/1(fqs) -> Subsistema electromagnético/1(v_qs^r)
  Tº_amb/1 -> Subsistema térmico/4(Tº_amb)
  Mux/1 -> i_abcs/1
  TI_PARK/1(fas) -> Mux/1
  TI_PARK/2(fbs) -> Mux/2
  TI_PARK/3(fcs) -> Mux/3
  v_as/1 -> TD_PARK/1(fas)
  v_cs/1 -> TD_PARK/3(fcs)
  Gain/1 -> TI_PARK/4(theta_r), TD_PARK/4(theta_r)
  v_bs/1 -> TD_PARK/2(fbs)
  Gain1/1 -> Sin/1
  Sin/1 -> Gain2/1
  Gain2/1 -> Sum/1
  T_per/1 -> Sum/2
  TD_PARK/2(fds) -> Subsistema electromagnético/2(v_ds^r)
  TD_PARK/3(f0s) -> Subsistema electromagnético/3(v_0s)
  Subsistema térmico/1(r_s) -> Subsistema electromagnético/4(r_s)
  Subsistema térmico/2(T_s) -> T_s/1
  Subsistema mecánico completo/1(theta_m(t)) -> theta_m/1, Gain1/1, Gain/1

== system consigna_5_1/Sistema linealizado por retroalimentación no lineal6/Inversor: Modulador de tensión ==
  v_as* : Inport
  v_bs* : Inport  Port=2
  v_cs* : Inport  Port=3
  Gain5 : Gain
  Gain6 : Gain
  Gain7 : Gain
  v_as : Outport
  v_bs : Outport  Port=2
  v_cs : Outport  Port=3
  wires:
  v_as*/1 -> Gain5/1
  Gain5/1 -> v_as/1
  v_cs*/1 -> Gain7/1
  v_bs*/1 -> Gain6/1
  Gain7/1 -> v_cs/1
  Gain6/1 -> v_bs/1

== system consigna_5_1/Sistema linealizado por retroalimentación no lineal6/Subsistema físico no lineal ==
  note: Retroalimentación natural del torque gravitacional
  T_per : Inport
  v_as : Inport  Port=2
  v_bs : Inport  Port=3
  v_cs : Inport  Port=4
  Tº_amb : Inport  Port=5
  Gain : Gain  Gain=P_p
  Gain1 : Gain  Gain=1/r
  Gain2 : Gain  Gain=k_l
  Mux : Mux  Inputs=3
  Sin : Trigonometry
  Subsistema electromagnético : Subsystem
      settings: PortSchema="{\"entries\":[{\"content\":{\"sides\":[{\"content\":{\"connectorIds\":[\"In1\",\"In2\",\"In3\",\"In4\"]},\"type\":\"ConnectorPlacement.EquallySpacedRectSide\",\"uuid\":\"c9fae60f-a644-4c7d-9a50-e330e891aba8\"},{\"content\":{\"connectorIds\":[\"Out1\",\"Out2\",\"Out3\",\"Out4\"],\"side\":\"RIGHT\"},\"type\":\"ConnectorPlacement.EquallySpacedRectSide\",\"uuid\":\"1bd25713-f5e9-4106-83eb-fb9f8a30d88e\"},{\"content\":{\"connectorIds\":[\"In5\"],\"side\":\"TOP\"},\"type\":\"ConnectorPlacement.EquallySpacedRectSide\",\"uuid\":\"c2f005dd-e04f-426d-b804-ce475aa5422d\"}]},\"type\":\"ConnectorPlacement.EquallySpacedConnector\",\"uuid\":\"9bdc4406-fcef-47cb-a5c0-d4f33f547a91\"}],\"packageUris\":[\"http://schema.mathworks.com/mf0/Connector/R2020b\"],\"version\":\"1.0\"}"
  Subsistema mecánico completo : Subsystem
  Subsistema térmico : Subsystem
  Sum : Sum  Inputs=++|
  TD_PARK : MATLAB Function  TreatAsAtomicUnit=on
  TI_PARK : MATLAB Function  TreatAsAtomicUnit=on
  theta_m : Outport
  T_s : Outport  Port=2
  i_abcs : Outport  Port=3
  T_m : Outport  Port=4
  omega_m : Outport  Port=5
  wires:
  Subsistema electromagnético/4(T_m) -> T_m/1, Subsistema mecánico completo/1(T_m)
  Subsistema electromagnético/3(i_0s) -> Subsistema térmico/3(i_0s^r), TI_PARK/3(f0s)
  Subsistema mecánico completo/2(omega_m(t)) -> Subsistema electromagnético/5(omega_m), omega_m/1
  Subsistema electromagnético/1(i_qs^r) -> Subsistema térmico/1(i_qs^r), TI_PARK/1(fqs)
  Subsistema electromagnético/2(i_ds^r) -> Subsistema térmico/2(i_ds^r), TI_PARK/2(fds)
  Sum/1 -> Subsistema mecánico completo/2(T_l)  "T_l"
  TD_PARK/1(fqs) -> Subsistema electromagnético/1(v_qs^r)
  Subsistema mecánico completo/1(theta_m(t)) -> theta_m/1, Gain1/1, Gain/1
  Tº_amb/1 -> Subsistema térmico/4(Tº_amb)
  Mux/1 -> i_abcs/1
  TI_PARK/1(fas) -> Mux/1
  TI_PARK/2(fbs) -> Mux/2
  TI_PARK/3(fcs) -> Mux/3
  v_as/1 -> TD_PARK/1(fas)
  v_cs/1 -> TD_PARK/3(fcs)
  Gain/1 -> TI_PARK/4(theta_r), TD_PARK/4(theta_r)
  v_bs/1 -> TD_PARK/2(fbs)
  Gain1/1 -> Sin/1
  Sin/1 -> Gain2/1
  Gain2/1 -> Sum/1
  T_per/1 -> Sum/2
  TD_PARK/2(fds) -> Subsistema electromagnético/2(v_ds^r)
  TD_PARK/3(f0s) -> Subsistema electromagnético/3(v_0s)
  Subsistema térmico/1(r_s) -> Subsistema electromagnético/4(r_s)
  Subsistema térmico/2(T_s) -> T_s/1

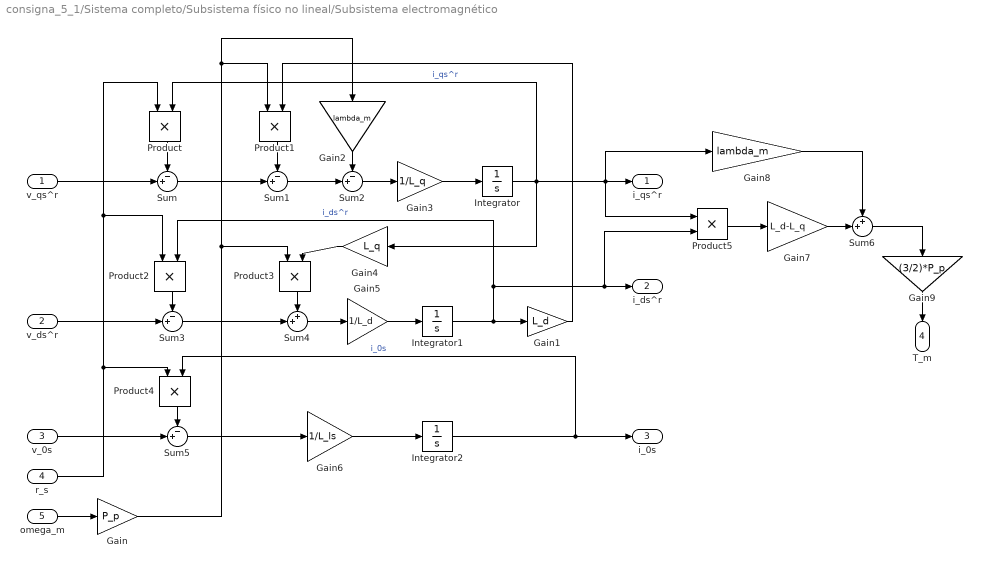
== system consigna_5_1/Sistema completo/Subsistema físico no lineal/Subsistema electromagnético ==
  v_qs^r : Inport
  v_ds^r : Inport  Port=2
  v_0s : Inport  Port=3
  r_s : Inport  Port=4
  omega_m : Inport  Port=5
  Gain : Gain  Gain=P_p
  Gain1 : Gain  Gain=L_d
  Gain2 : Gain  Gain=lambda_m
  Gain3 : Gain  Gain=1/L_q
  Gain4 : Gain  Gain=L_q
  Gain5 : Gain  Gain=1/L_d
  Gain6 : Gain  Gain=1/L_ls
  Gain7 : Gain  Gain=L_d-L_q
  Gain8 : Gain  Gain=lambda_m
  Gain9 : Gain  Gain=(3/2)*P_p
  Integrator : Integrator
  Integrator1 : Integrator
  Integrator2 : Integrator
  Product{,1..5} (6 alike) : Product
  Sum{,1..3,5} (5 alike) : Sum  Inputs=-+|
  Sum4 : Sum  Inputs=++|
  Sum6 : Sum  Inputs=++|
  i_qs^r : Outport
  i_ds^r : Outport  Port=2
  i_0s : Outport  Port=3
  T_m : Outport  Port=4
  wires:
  v_qs^r/1 -> Sum/2
  Product/1 -> Sum/1
  Sum/1 -> Sum1/2
  Integrator/1 -> Gain8/1, Product5/1, i_qs^r/1, Product/2, Gain4/1  "i_qs^r"
  omega_m/1 -> Gain/1
  Gain/1 -> Gain2/1, Product1/1, Product3/1
  Integrator1/1 -> Product2/2, Product5/2, i_ds^r/1, Gain1/1  "i_ds^r"
  Gain1/1 -> Product1/2
  Sum1/1 -> Sum2/2
  Sum2/1 -> Gain3/1
  Gain2/1 -> Sum2/1
  Product1/1 -> Sum1/1
  Gain3/1 -> Integrator/1
  Product2/1 -> Sum3/1
  v_ds^r/1 -> Sum3/2
  Sum3/1 -> Sum4/2
  Product3/1 -> Sum4/1
  Gain4/1 -> Product3/2
  Gain5/1 -> Integrator1/1
  Sum4/1 -> Gain5/1
  Integrator2/1 -> Product4/2, i_0s/1  "i_0s"
  r_s/1 -> Product4/1, Product/1, Product2/1
  Product4/1 -> Sum5/1
  v_0s/1 -> Sum5/2
  Sum5/1 -> Gain6/1
  Gain6/1 -> Integrator2/1
  Product5/1 -> Gain7/1
  Gain7/1 -> Sum6/2
  Gain8/1 -> Sum6/1
  Sum6/1 -> Gain9/1
  Gain9/1 -> T_m/1

== system consigna_5_1/Sistema completo/Subsistema físico no lineal/Subsistema mecánico completo ==
  T_m : Inport
  T_l : Inport  Port=2
  Gain : Gain  Gain=b_m + b_l / (r^2)
  Gain1 : Gain  Gain=1/r
  Gain2 : Gain  Gain=1/(J_m + J_l / r^2)
  Sum : Sum  Inputs=-+-
  omega_m(0) = 0 : Integrator
  theta_m(0) = 0 : Integrator
  theta_m(t) : Outport
  omega_m(t) : Outport  Port=2
  wires:
  Gain2/1 -> omega_m(0) = 0/1  "domega_m(t)/dt"
  Gain1/1 -> Sum/1
  theta_m(0) = 0/1 -> theta_m(t)/1  "theta_m(t)"
  omega_m(0) = 0/1 -> omega_m(t)/1, Gain/1, theta_m(0) = 0/1  "omega_m(t)"
  Sum/1 -> Gain2/1
  Gain/1 -> Sum/3
  T_l/1 -> Gain1/1
  T_m/1 -> Sum/2

== system consigna_5_1/Sistema completo/Subsistema físico no lineal/Subsistema térmico ==
  i_qs^r : Inport
  i_ds^r : Inport  Port=2
  i_0s^r : Inport  Port=3
  Tº_amb : Inport  Port=4
  Constant : Constant  Value=Temp_s_ref
  Constant1 : Constant
  Gain : Gain  Gain=1/C_ts
  Gain1 : Gain  Gain=3/2
  Gain2 : Gain  Gain=1/R_ts_amb
  Gain3 : Gain  Gain=alpha_cu
  Gain4 : Gain  Gain=R_s_40
  Gain5 : Gain  Gain=2
  Integrator : Integrator  InitialCondition=40
  Product : Product
  Square : Math  Operator=square
  Square1 : Math  Operator=square
  Square2 : Math  Operator=square
  Sum : Sum  Inputs=+++
  Sum1 : Sum  Inputs=-|+
  Sum2 : Sum  Inputs=|+-
  Sum3 : Sum  Inputs=|+-
  Sum4 : Sum  Inputs=|++
  r_s : Outport
  T_s : Outport  Port=2
  wires:
  i_qs^r/1 -> Square/1
  i_ds^r/1 -> Square1/1
  i_0s^r/1 -> Square2/1
  Gain/1 -> Integrator/1
  Square/1 -> Sum/1
  Square1/1 -> Sum/2
  Square2/1 -> Gain5/1
  Sum/1 -> Product/1
  Product/1 -> Gain1/1
  Tº_amb/1 -> Sum1/1
  Integrator/1 -> T_s/1, Sum3/1, Sum1/2
  Sum1/1 -> Gain2/1
  Gain1/1 -> Sum2/1
  Gain2/1 -> Sum2/2
  Sum2/1 -> Gain/1
  Constant/1 -> Sum3/2
  Sum3/1 -> Gain3/1
  Gain3/1 -> Sum4/1
  Constant1/1 -> Sum4/2
  Sum4/1 -> Gain4/1
  Gain4/1 -> Product/2, r_s/1
  Gain5/1 -> Sum/3

== system consigna_5_1/Sistema linealizado por retroalimentación no lineal1/Subsistema físico no lineal/Subsistema electromagnético ==
  v_qs^r : Inport
  v_ds^r : Inport  Port=2
  v_0s : Inport  Port=3
  r_s : Inport  Port=4
  omega_m : Inport  Port=5
  Gain : Gain  Gain=P_p
  Gain1 : Gain  Gain=L_d
  Gain2 : Gain  Gain=lambda_m
  Gain3 : Gain  Gain=1/L_q
  Gain4 : Gain  Gain=L_q
  Gain5 : Gain  Gain=1/L_d
  Gain6 : Gain  Gain=1/L_ls
  Gain7 : Gain  Gain=L_d-L_q
  Gain8 : Gain  Gain=lambda_m
  Gain9 : Gain  Gain=(3/2)*P_p
  Integrator : Integrator
  Integrator1 : Integrator
  Integrator2 : Integrator
  Product{,1..5} (6 alike) : Product
  Sum{,1..3,5} (5 alike) : Sum  Inputs=-+|
  Sum4 : Sum  Inputs=++|
  Sum6 : Sum  Inputs=++|
  i_qs^r : Outport
  i_ds^r : Outport  Port=2
  i_0s : Outport  Port=3
  T_m : Outport  Port=4
  wires:
  v_qs^r/1 -> Sum/2
  Product/1 -> Sum/1
  Sum/1 -> Sum1/2
  Integrator/1 -> Gain8/1, Product5/1, i_qs^r/1, Product/2, Gain4/1  "i_qs^r"
  omega_m/1 -> Gain/1
  Gain/1 -> Gain2/1, Product1/1, Product3/1
  Integrator1/1 -> Product2/2, Product5/2, i_ds^r/1, Gain1/1  "i_ds^r"
  Gain1/1 -> Product1/2
  Sum1/1 -> Sum2/2
  Sum2/1 -> Gain3/1
  Gain2/1 -> Sum2/1
  Product1/1 -> Sum1/1
  Gain3/1 -> Integrator/1
  Product2/1 -> Sum3/1
  v_ds^r/1 -> Sum3/2
  Sum3/1 -> Sum4/2
  Product3/1 -> Sum4/1
  Gain4/1 -> Product3/2
  Gain5/1 -> Integrator1/1
  Sum4/1 -> Gain5/1
  Integrator2/1 -> Product4/2, i_0s/1  "i_0s"
  r_s/1 -> Product4/1, Product/1, Product2/1
  Product4/1 -> Sum5/1
  v_0s/1 -> Sum5/2
  Sum5/1 -> Gain6/1
  Gain6/1 -> Integrator2/1
  Product5/1 -> Gain7/1
  Gain7/1 -> Sum6/2
  Gain8/1 -> Sum6/1
  Sum6/1 -> Gain9/1
  Gain9/1 -> T_m/1

== system consigna_5_1/Sistema linealizado por retroalimentación no lineal1/Subsistema físico no lineal/Subsistema mecánico completo ==
  T_m : Inport
  T_l : Inport  Port=2
  Gain : Gain  Gain=b_m + b_l / (r^2)
  Gain1 : Gain  Gain=1/r
  Gain2 : Gain  Gain=1/(J_m + J_l / r^2)
  Sum : Sum  Inputs=-+-
  omega_m(0) = 0 : Integrator
  theta_m(0) = 0 : Integrator
  theta_m(t) : Outport
  omega_m(t) : Outport  Port=2
  wires:
  Gain2/1 -> omega_m(0) = 0/1  "domega_m(t)/dt"
  Gain1/1 -> Sum/1
  theta_m(0) = 0/1 -> theta_m(t)/1  "theta_m(t)"
  omega_m(0) = 0/1 -> omega_m(t)/1, Gain/1, theta_m(0) = 0/1  "omega_m(t)"
  Sum/1 -> Gain2/1
  Gain/1 -> Sum/3
  T_l/1 -> Gain1/1
  T_m/1 -> Sum/2

== system consigna_5_1/Sistema linealizado por retroalimentación no lineal1/Subsistema físico no lineal/Subsistema térmico ==
  i_qs^r : Inport
  i_ds^r : Inport  Port=2
  i_0s^r : Inport  Port=3
  Tº_amb : Inport  Port=4
  Constant : Constant  Value=Temp_s_ref
  Constant1 : Constant
  Gain : Gain  Gain=1/C_ts
  Gain1 : Gain  Gain=3/2
  Gain2 : Gain  Gain=1/R_ts_amb
  Gain3 : Gain  Gain=alpha_cu
  Gain4 : Gain  Gain=R_s_40
  Gain5 : Gain  Gain=2
  Integrator : Integrator  InitialCondition=40
  Product : Product
  Square : Math  Operator=square
  Square1 : Math  Operator=square
  Square2 : Math  Operator=square
  Sum : Sum  Inputs=+++
  Sum1 : Sum  Inputs=-|+
  Sum2 : Sum  Inputs=|+-
  Sum3 : Sum  Inputs=|+-
  Sum4 : Sum  Inputs=|++
  r_s : Outport
  T_s : Outport  Port=2
  wires:
  i_qs^r/1 -> Square/1
  i_ds^r/1 -> Square1/1
  i_0s^r/1 -> Square2/1
  Gain/1 -> Integrator/1
  Square/1 -> Sum/1
  Square1/1 -> Sum/2
  Sum/1 -> Product/1
  Product/1 -> Gain1/1
  Tº_amb/1 -> Sum1/1
  Integrator/1 -> T_s/1, Sum3/1, Sum1/2
  Sum1/1 -> Gain2/1
  Gain1/1 -> Sum2/1
  Gain2/1 -> Sum2/2
  Sum2/1 -> Gain/1
  Constant/1 -> Sum3/2
  Sum3/1 -> Gain3/1
  Gain3/1 -> Sum4/1
  Constant1/1 -> Sum4/2
  Sum4/1 -> Gain4/1
  Gain4/1 -> Product/2, r_s/1
  Square2/1 -> Gain5/1
  Gain5/1 -> Sum/3

== system consigna_5_1/Sistema linealizado por retroalimentación no lineal2/Subsistema físico no lineal/Subsistema electromagnético ==
  v_qs^r : Inport
  v_ds^r : Inport  Port=2
  v_0s : Inport  Port=3
  r_s : Inport  Port=4
  omega_m : Inport  Port=5
  Gain : Gain  Gain=P_p
  Gain1 : Gain  Gain=L_d
  Gain2 : Gain  Gain=lambda_m
  Gain3 : Gain  Gain=1/L_q
  Gain4 : Gain  Gain=L_q
  Gain5 : Gain  Gain=1/L_d
  Gain6 : Gain  Gain=1/L_ls
  Gain7 : Gain  Gain=L_d-L_q
  Gain8 : Gain  Gain=lambda_m
  Gain9 : Gain  Gain=(3/2)*P_p
  Integrator : Integrator
  Integrator1 : Integrator  InitialCondition=0.5
  Integrator2 : Integrator
  Product{,1..5} (6 alike) : Product
  Sum{,1..3,5} (5 alike) : Sum  Inputs=-+|
  Sum4 : Sum  Inputs=++|
  Sum6 : Sum  Inputs=++|
  i_qs^r : Outport
  i_ds^r : Outport  Port=2
  i_0s : Outport  Port=3
  T_m : Outport  Port=4
  wires:
  v_qs^r/1 -> Sum/2
  Product/1 -> Sum/1
  Sum/1 -> Sum1/2
  Integrator/1 -> Gain8/1, Product5/1, i_qs^r/1, Product/2, Gain4/1  "i_qs^r"
  omega_m/1 -> Gain/1
  Gain/1 -> Gain2/1, Product1/1, Product3/1
  Integrator1/1 -> Product2/2, Product5/2, i_ds^r/1, Gain1/1  "i_ds^r"
  Gain1/1 -> Product1/2
  Sum1/1 -> Sum2/2
  Sum2/1 -> Gain3/1
  Gain2/1 -> Sum2/1
  Product1/1 -> Sum1/1
  Gain3/1 -> Integrator/1
  Product2/1 -> Sum3/1
  v_ds^r/1 -> Sum3/2
  Sum3/1 -> Sum4/2
  Product3/1 -> Sum4/1
  Gain4/1 -> Product3/2
  Gain5/1 -> Integrator1/1
  Sum4/1 -> Gain5/1
  Integrator2/1 -> Product4/2, i_0s/1  "i_0s"
  r_s/1 -> Product4/1, Product/1, Product2/1
  Product4/1 -> Sum5/1
  v_0s/1 -> Sum5/2
  Sum5/1 -> Gain6/1
  Gain6/1 -> Integrator2/1
  Product5/1 -> Gain7/1
  Gain7/1 -> Sum6/2
  Gain8/1 -> Sum6/1
  Sum6/1 -> Gain9/1
  Gain9/1 -> T_m/1

== system consigna_5_1/Sistema linealizado por retroalimentación no lineal2/Subsistema físico no lineal/Subsistema mecánico completo ==
  T_m : Inport
  T_l : Inport  Port=2
  Gain : Gain  Gain=b_m + b_l / (r^2)
  Gain1 : Gain  Gain=1/r
  Gain2 : Gain  Gain=1/(J_m + J_l / r^2)
  Sum : Sum  Inputs=-+-
  omega_m(0) = 0 : Integrator
  theta_m(0) = 0 : Integrator
  theta_m(t) : Outport
  omega_m(t) : Outport  Port=2
  wires:
  Gain2/1 -> omega_m(0) = 0/1  "domega_m(t)/dt"
  Gain1/1 -> Sum/1
  theta_m(0) = 0/1 -> theta_m(t)/1  "theta_m(t)"
  omega_m(0) = 0/1 -> omega_m(t)/1, Gain/1, theta_m(0) = 0/1  "omega_m(t)"
  Sum/1 -> Gain2/1
  Gain/1 -> Sum/3
  T_l/1 -> Gain1/1
  T_m/1 -> Sum/2

== system consigna_5_1/Sistema linealizado por retroalimentación no lineal2/Subsistema físico no lineal/Subsistema térmico ==
  i_qs^r : Inport
  i_ds^r : Inport  Port=2
  i_0s^r : Inport  Port=3
  Tº_amb : Inport  Port=4
  Constant : Constant  Value=Temp_s_ref
  Constant1 : Constant
  Gain : Gain  Gain=1/C_ts
  Gain1 : Gain  Gain=3/2
  Gain2 : Gain  Gain=1/R_ts_amb
  Gain3 : Gain  Gain=alpha_cu
  Gain4 : Gain  Gain=R_s_40
  Gain5 : Gain  Gain=2
  Integrator : Integrator  InitialCondition=40
  Product : Product
  Square : Math  Operator=square
  Square1 : Math  Operator=square
  Square2 : Math  Operator=square
  Sum : Sum  Inputs=+++
  Sum1 : Sum  Inputs=-|+
  Sum2 : Sum  Inputs=|+-
  Sum3 : Sum  Inputs=|+-
  Sum4 : Sum  Inputs=|++
  r_s : Outport
  T_s : Outport  Port=2
  wires:
  i_qs^r/1 -> Square/1
  i_ds^r/1 -> Square1/1
  i_0s^r/1 -> Square2/1
  Gain/1 -> Integrator/1
  Square/1 -> Sum/1
  Square1/1 -> Sum/2
  Sum/1 -> Product/1
  Product/1 -> Gain1/1
  Tº_amb/1 -> Sum1/1
  Integrator/1 -> T_s/1, Sum3/1, Sum1/2
  Sum1/1 -> Gain2/1
  Gain1/1 -> Sum2/1
  Gain2/1 -> Sum2/2
  Sum2/1 -> Gain/1
  Constant/1 -> Sum3/2
  Sum3/1 -> Gain3/1
  Gain3/1 -> Sum4/1
  Constant1/1 -> Sum4/2
  Sum4/1 -> Gain4/1
  Gain4/1 -> Product/2, r_s/1
  Square2/1 -> Gain5/1
  Gain5/1 -> Sum/3

== system consigna_5_1/Sistema linealizado por retroalimentación no lineal3/Subsistema físico no lineal/Subsistema electromagnético ==
  v_qs^r : Inport
  v_ds^r : Inport  Port=2
  v_0s : Inport  Port=3
  r_s : Inport  Port=4
  omega_m : Inport  Port=5
  Gain : Gain  Gain=P_p
  Gain1 : Gain  Gain=L_d
  Gain2 : Gain  Gain=lambda_m
  Gain3 : Gain  Gain=1/L_q
  Gain4 : Gain  Gain=L_q
  Gain5 : Gain  Gain=1/L_d
  Gain6 : Gain  Gain=1/L_ls
  Gain7 : Gain  Gain=L_d-L_q
  Gain8 : Gain  Gain=lambda_m
  Gain9 : Gain  Gain=(3/2)*P_p
  Integrator : Integrator
  Integrator1 : Integrator  InitialCondition=-0.5
  Integrator2 : Integrator
  Product{,1..5} (6 alike) : Product
  Sum{,1..3,5} (5 alike) : Sum  Inputs=-+|
  Sum4 : Sum  Inputs=++|
  Sum6 : Sum  Inputs=++|
  i_qs^r : Outport
  i_ds^r : Outport  Port=2
  i_0s : Outport  Port=3
  T_m : Outport  Port=4
  wires:
  v_qs^r/1 -> Sum/2
  Product/1 -> Sum/1
  Sum/1 -> Sum1/2
  Integrator/1 -> Gain8/1, Product5/1, i_qs^r/1, Product/2, Gain4/1  "i_qs^r"
  omega_m/1 -> Gain/1
  Gain/1 -> Gain2/1, Product1/1, Product3/1
  Integrator1/1 -> Product2/2, Product5/2, i_ds^r/1, Gain1/1  "i_ds^r"
  Gain1/1 -> Product1/2
  Sum1/1 -> Sum2/2
  Sum2/1 -> Gain3/1
  Gain2/1 -> Sum2/1
  Product1/1 -> Sum1/1
  Gain3/1 -> Integrator/1
  Product2/1 -> Sum3/1
  v_ds^r/1 -> Sum3/2
  Sum3/1 -> Sum4/2
  Product3/1 -> Sum4/1
  Gain4/1 -> Product3/2
  Gain5/1 -> Integrator1/1
  Sum4/1 -> Gain5/1
  Integrator2/1 -> Product4/2, i_0s/1  "i_0s"
  r_s/1 -> Product4/1, Product/1, Product2/1
  Product4/1 -> Sum5/1
  v_0s/1 -> Sum5/2
  Sum5/1 -> Gain6/1
  Gain6/1 -> Integrator2/1
  Product5/1 -> Gain7/1
  Gain7/1 -> Sum6/2
  Gain8/1 -> Sum6/1
  Sum6/1 -> Gain9/1
  Gain9/1 -> T_m/1

== system consigna_5_1/Sistema linealizado por retroalimentación no lineal3/Subsistema físico no lineal/Subsistema mecánico completo ==
  T_m : Inport
  T_l : Inport  Port=2
  Gain : Gain  Gain=b_m + b_l / (r^2)
  Gain1 : Gain  Gain=1/r
  Gain2 : Gain  Gain=1/(J_m + J_l / r^2)
  Sum : Sum  Inputs=-+-
  omega_m(0) = 0 : Integrator
  theta_m(0) = 0 : Integrator
  theta_m(t) : Outport
  omega_m(t) : Outport  Port=2
  wires:
  Gain2/1 -> omega_m(0) = 0/1  "domega_m(t)/dt"
  Gain1/1 -> Sum/1
  theta_m(0) = 0/1 -> theta_m(t)/1  "theta_m(t)"
  omega_m(0) = 0/1 -> omega_m(t)/1, Gain/1, theta_m(0) = 0/1  "omega_m(t)"
  Sum/1 -> Gain2/1
  Gain/1 -> Sum/3
  T_l/1 -> Gain1/1
  T_m/1 -> Sum/2

== system consigna_5_1/Sistema linealizado por retroalimentación no lineal3/Subsistema físico no lineal/Subsistema térmico ==
  i_qs^r : Inport
  i_ds^r : Inport  Port=2
  i_0s^r : Inport  Port=3
  Tº_amb : Inport  Port=4
  Constant : Constant  Value=Temp_s_ref
  Constant1 : Constant
  Gain : Gain  Gain=1/C_ts
  Gain1 : Gain  Gain=3/2
  Gain2 : Gain  Gain=1/R_ts_amb
  Gain3 : Gain  Gain=alpha_cu
  Gain4 : Gain  Gain=R_s_40
  Gain5 : Gain  Gain=2
  Integrator : Integrator  InitialCondition=40
  Product : Product
  Square : Math  Operator=square
  Square1 : Math  Operator=square
  Square2 : Math  Operator=square
  Sum : Sum  Inputs=+++
  Sum1 : Sum  Inputs=-|+
  Sum2 : Sum  Inputs=|+-
  Sum3 : Sum  Inputs=|+-
  Sum4 : Sum  Inputs=|++
  r_s : Outport
  T_s : Outport  Port=2
  wires:
  i_qs^r/1 -> Square/1
  i_ds^r/1 -> Square1/1
  i_0s^r/1 -> Square2/1
  Gain/1 -> Integrator/1
  Square/1 -> Sum/1
  Square1/1 -> Sum/2
  Sum/1 -> Product/1
  Product/1 -> Gain1/1
  Tº_amb/1 -> Sum1/1
  Integrator/1 -> T_s/1, Sum3/1, Sum1/2
  Sum1/1 -> Gain2/1
  Gain1/1 -> Sum2/1
  Gain2/1 -> Sum2/2
  Sum2/1 -> Gain/1
  Constant/1 -> Sum3/2
  Sum3/1 -> Gain3/1
  Gain3/1 -> Sum4/1
  Constant1/1 -> Sum4/2
  Sum4/1 -> Gain4/1
  Gain4/1 -> Product/2, r_s/1
  Square2/1 -> Gain5/1
  Gain5/1 -> Sum/3

== system consigna_5_1/Sistema linealizado por retroalimentación no lineal4/Subsistema físico no lineal/Subsistema electromagnético ==
  v_qs^r : Inport
  v_ds^r : Inport  Port=2
  v_0s : Inport  Port=3
  r_s : Inport  Port=4
  omega_m : Inport  Port=5
  Gain : Gain  Gain=P_p
  Gain1 : Gain  Gain=L_d
  Gain2 : Gain  Gain=lambda_m
  Gain3 : Gain  Gain=1/L_q
  Gain4 : Gain  Gain=L_q
  Gain5 : Gain  Gain=1/L_d
  Gain6 : Gain  Gain=1/L_ls
  Gain7 : Gain  Gain=L_d-L_q
  Gain8 : Gain  Gain=lambda_m
  Gain9 : Gain  Gain=(3/2)*P_p
  Integrator : Integrator
  Integrator1 : Integrator
  Integrator2 : Integrator
  Product{,1..5} (6 alike) : Product
  Sum{,1..3,5} (5 alike) : Sum  Inputs=-+|
  Sum4 : Sum  Inputs=++|
  Sum6 : Sum  Inputs=++|
  i_qs^r : Outport
  i_ds^r : Outport  Port=2
  i_0s : Outport  Port=3
  T_m : Outport  Port=4
  wires:
  v_qs^r/1 -> Sum/2
  Product/1 -> Sum/1
  Sum/1 -> Sum1/2
  Integrator/1 -> Gain8/1, Product5/1, i_qs^r/1, Product/2, Gain4/1  "i_qs^r"
  omega_m/1 -> Gain/1
  Gain/1 -> Gain2/1, Product1/1, Product3/1
  Integrator1/1 -> Product2/2, Product5/2, i_ds^r/1, Gain1/1  "i_ds^r"
  Gain1/1 -> Product1/2
  Sum1/1 -> Sum2/2
  Sum2/1 -> Gain3/1
  Gain2/1 -> Sum2/1
  Product1/1 -> Sum1/1
  Gain3/1 -> Integrator/1
  Product2/1 -> Sum3/1
  v_ds^r/1 -> Sum3/2
  Sum3/1 -> Sum4/2
  Product3/1 -> Sum4/1
  Gain4/1 -> Product3/2
  Gain5/1 -> Integrator1/1
  Sum4/1 -> Gain5/1
  Integrator2/1 -> Product4/2, i_0s/1  "i_0s"
  r_s/1 -> Product4/1, Product/1, Product2/1
  Product4/1 -> Sum5/1
  v_0s/1 -> Sum5/2
  Sum5/1 -> Gain6/1
  Gain6/1 -> Integrator2/1
  Product5/1 -> Gain7/1
  Gain7/1 -> Sum6/2
  Gain8/1 -> Sum6/1
  Sum6/1 -> Gain9/1
  Gain9/1 -> T_m/1

== system consigna_5_1/Sistema linealizado por retroalimentación no lineal4/Subsistema físico no lineal/Subsistema mecánico completo ==
  T_m : Inport
  T_l : Inport  Port=2
  Gain : Gain  Gain=b_m + b_l / (r^2)
  Gain1 : Gain  Gain=1/r
  Gain2 : Gain  Gain=1/(J_m + J_l / r^2)
  Sum : Sum  Inputs=-+-
  omega_m(0) = 0 : Integrator
  theta_m(0) = 0 : Integrator
  theta_m(t) : Outport
  omega_m(t) : Outport  Port=2
  wires:
  Gain2/1 -> omega_m(0) = 0/1  "domega_m(t)/dt"
  Gain1/1 -> Sum/1
  theta_m(0) = 0/1 -> theta_m(t)/1  "theta_m(t)"
  omega_m(0) = 0/1 -> omega_m(t)/1, Gain/1, theta_m(0) = 0/1  "omega_m(t)"
  Sum/1 -> Gain2/1
  Gain/1 -> Sum/3
  T_l/1 -> Gain1/1
  T_m/1 -> Sum/2

== system consigna_5_1/Sistema linealizado por retroalimentación no lineal4/Subsistema físico no lineal/Subsistema térmico ==
  i_qs^r : Inport
  i_ds^r : Inport  Port=2
  i_0s^r : Inport  Port=3
  Tº_amb : Inport  Port=4
  Constant : Constant  Value=Temp_s_ref
  Constant1 : Constant
  Gain : Gain  Gain=1/C_ts
  Gain1 : Gain  Gain=3/2
  Gain2 : Gain  Gain=1/R_ts_amb
  Gain3 : Gain  Gain=alpha_cu
  Gain4 : Gain  Gain=R_s_40
  Gain5 : Gain  Gain=2
  Integrator : Integrator  InitialCondition=40
  Product : Product
  Square : Math  Operator=square
  Square1 : Math  Operator=square
  Square2 : Math  Operator=square
  Sum : Sum  Inputs=+++
  Sum1 : Sum  Inputs=-|+
  Sum2 : Sum  Inputs=|+-
  Sum3 : Sum  Inputs=|+-
  Sum4 : Sum  Inputs=|++
  r_s : Outport
  T_s : Outport  Port=2
  wires:
  i_qs^r/1 -> Square/1
  i_ds^r/1 -> Square1/1
  i_0s^r/1 -> Square2/1
  Gain/1 -> Integrator/1
  Square/1 -> Sum/1
  Square1/1 -> Sum/2
  Sum/1 -> Product/1
  Product/1 -> Gain1/1
  Tº_amb/1 -> Sum1/1
  Integrator/1 -> T_s/1, Sum3/1, Sum1/2
  Sum1/1 -> Gain2/1
  Gain1/1 -> Sum2/1
  Gain2/1 -> Sum2/2
  Sum2/1 -> Gain/1
  Constant/1 -> Sum3/2
  Sum3/1 -> Gain3/1
  Gain3/1 -> Sum4/1
  Constant1/1 -> Sum4/2
  Sum4/1 -> Gain4/1
  Gain4/1 -> Product/2, r_s/1
  Square2/1 -> Gain5/1
  Gain5/1 -> Sum/3

== system consigna_5_1/Sistema linealizado por retroalimentación no lineal5/Subsistema físico no lineal/Subsistema electromagnético ==
  v_qs^r : Inport
  v_ds^r : Inport  Port=2
  v_0s : Inport  Port=3
  r_s : Inport  Port=4
  omega_m : Inport  Port=5
  Gain : Gain  Gain=P_p
  Gain1 : Gain  Gain=L_d
  Gain2 : Gain  Gain=lambda_m
  Gain3 : Gain  Gain=1/L_q
  Gain4 : Gain  Gain=L_q
  Gain5 : Gain  Gain=1/L_d
  Gain6 : Gain  Gain=1/L_ls
  Gain7 : Gain  Gain=L_d-L_q
  Gain8 : Gain  Gain=lambda_m
  Gain9 : Gain  Gain=(3/2)*P_p
  Integrator : Integrator
  Integrator1 : Integrator
  Integrator2 : Integrator
  Product{,1..5} (6 alike) : Product
  Sum{,1..3,5} (5 alike) : Sum  Inputs=-+|
  Sum4 : Sum  Inputs=++|
  Sum6 : Sum  Inputs=++|
  i_qs^r : Outport
  i_ds^r : Outport  Port=2
  i_0s : Outport  Port=3
  T_m : Outport  Port=4
  wires:
  v_qs^r/1 -> Sum/2
  Product/1 -> Sum/1
  Sum/1 -> Sum1/2
  Integrator/1 -> Gain8/1, Product5/1, i_qs^r/1, Product/2, Gain4/1  "i_qs^r"
  omega_m/1 -> Gain/1
  Gain/1 -> Gain2/1, Product1/1, Product3/1
  Integrator1/1 -> Product2/2, Product5/2, i_ds^r/1, Gain1/1  "i_ds^r"
  Gain1/1 -> Product1/2
  Sum1/1 -> Sum2/2
  Sum2/1 -> Gain3/1
  Gain2/1 -> Sum2/1
  Product1/1 -> Sum1/1
  Gain3/1 -> Integrator/1
  Product2/1 -> Sum3/1
  v_ds^r/1 -> Sum3/2
  Sum3/1 -> Sum4/2
  Product3/1 -> Sum4/1
  Gain4/1 -> Product3/2
  Gain5/1 -> Integrator1/1
  Sum4/1 -> Gain5/1
  Integrator2/1 -> Product4/2, i_0s/1  "i_0s"
  r_s/1 -> Product4/1, Product/1, Product2/1
  Product4/1 -> Sum5/1
  v_0s/1 -> Sum5/2
  Sum5/1 -> Gain6/1
  Gain6/1 -> Integrator2/1
  Product5/1 -> Gain7/1
  Gain7/1 -> Sum6/2
  Gain8/1 -> Sum6/1
  Sum6/1 -> Gain9/1
  Gain9/1 -> T_m/1
